simulink library "csu_swm_switch_state_model_lib"  (R2014b)
settings: Solver=ode45  StartTime=0.0  StopTime=10.0  RelTol=1e-3
libraries: util_info_lib x1
settings Model: Creator=Nilesh  LastModifiedBy=mstewart

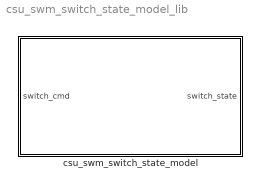
== system csu_swm_switch_state_model_lib ==
  csu_swm_switch_state_model : Subsystem  mask{switch_idx=0, num_switches=[]}
      mask prompts: switch_idx "Switch ID Number"; num_switches "Total number of switches"

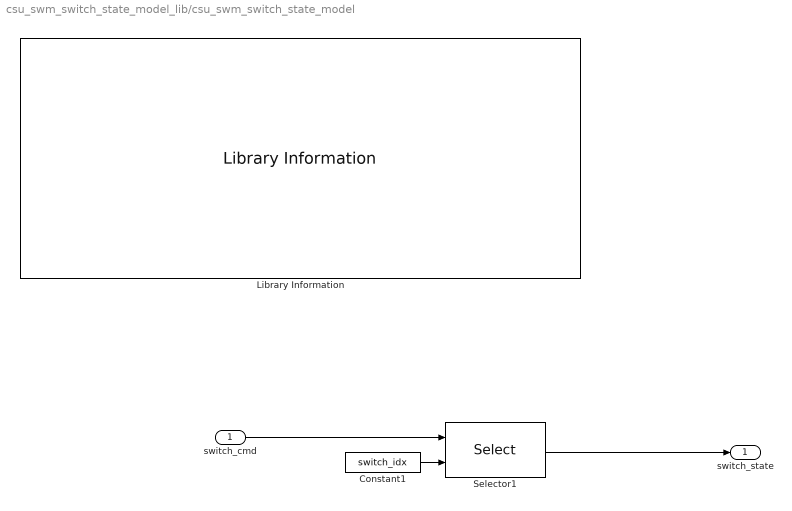
== system csu_swm_switch_state_model_lib/csu_swm_switch_state_model ==
  switch_cmd : Inport
  Constant1 : Constant  Value=switch_idx  OutDataTypeStr=uint8
  Library Information : util_info_lib/Library Information  owner='escrane'
  Selector1 : Selector  InputPortWidth=num_switches  IndexOptions=Index vector (port)  Indices=[1 3]
  switch_state : Outport
  wires:
  Constant1/1 -> Selector1/2
  switch_cmd/1 -> Selector1/1
  Selector1/1 -> switch_state/1
